simulink model "dyno"  (R2017a)
settings: Solver=FixedStepDiscrete  StartTime=0.0  StopTime=0.01  FixedStep=abs(Ts)  RelTol=1e-3
values from neighbouring files (symbols this model uses):
  Ts = 1    [dynorun.m]
undefined symbols (not defined in the file or in its folder): request, speed
libraries: elvio x5
settings Model: Creator=tstef  LastModifiedBy=elts2

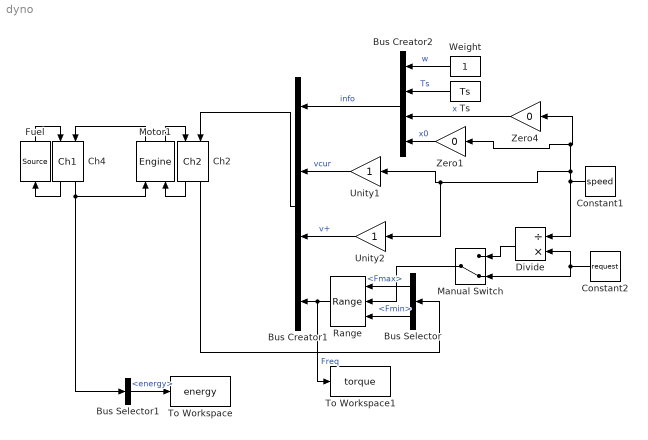
== system dyno ==
  Bus Creator1 : BusCreator  Inputs=4
  Bus Creator2 : BusCreator  Inputs=4
  Bus Selector : BusSelector  OutputSignals=Fmax,Fmin
  Bus Selector1 : BusSelector  OutputSignals=energy
  Ch2 : elvio/Basics/Ch2
  Ch4 : elvio/Basics/Ch1
  Constant1 : Constant  Value=speed
  Constant2 : Constant  Value=request
  Divide : Product  Inputs=/*
  Fuel : elvio/Basics/Source
  Manual Switch : ManualSwitch  CurrentSetting=0
  Motor1 : elvio/Drive/Engine  Tmax=60  Tmin=0  Tfrict=1  Ploss=100  lossf=0.01  lossnorm=1e6  lossR=0.1
  Range : elvio/Utilities/Range
  To Workspace : ToWorkspace  VariableName=energy  SampleTime=-1
      settings: MaxDataPoints=1
  To Workspace1 : ToWorkspace  VariableName=torque  SampleTime=-1
      settings: MaxDataPoints=1
  Ts : Constant  Value=Ts
  Unity1 : Gain
  Unity2 : Gain
  Weight : Constant
  Zero1 : Gain  Gain=0
  Zero4 : Gain  Gain=0
  wires:
  Motor1/1 -> Ch4/2
  Fuel/1 -> Ch4/1
  Ch4/1 -> Fuel/1
  Motor1/2 -> Ch2/1
  Constant1/1 -> Zero4/1, Zero1/1, Unity2/1, Unity1/1, Divide/1
  Unity1/1 -> Bus Creator1/2  "vcur"
  Bus Selector/1 -> Range/1  "<Fmax>"
  Zero1/1 -> Bus Creator2/4  "x0"
  Range/1 -> To Workspace1/1, Bus Creator1/4  "Freq"
  Zero4/1 -> Bus Creator2/3  "x"
  Bus Creator2/1 -> Bus Creator1/1  "info"
  Bus Selector/2 -> Range/3  "<Fmin>"
  Unity2/1 -> Bus Creator1/3  "v+"
  Ts/1 -> Bus Creator2/2  "Ts"
  Ch2/1 -> Motor1/2
  Bus Creator1/1 -> Ch2/2
  Ch2/2 -> Bus Selector/1
  Weight/1 -> Bus Creator2/1  "w"
  Manual Switch/1 -> Range/2
  Constant2/1 -> Manual Switch/2, Divide/2
  Divide/1 -> Manual Switch/1
  Bus Selector1/1 -> To Workspace/1  "<energy>"
  Ch4/2 -> Motor1/1, Bus Selector1/1
